simulink model "gm_sampleModel2027_3_sub_sub"  (R2023a)
settings: Solver=VariableStepAuto  StartTime=0.0  StopTime=10.0  RelTol=1e-3
libraries: hdlsllib x5, simulink x2
settings Model: Creator=user1  LastModifiedBy=user1
settings OptimizationCC: BlockReduction=off  ConditionallyExecuteInputs=off
settings DebuggingCC: InheritedTsInSrcMsg=none

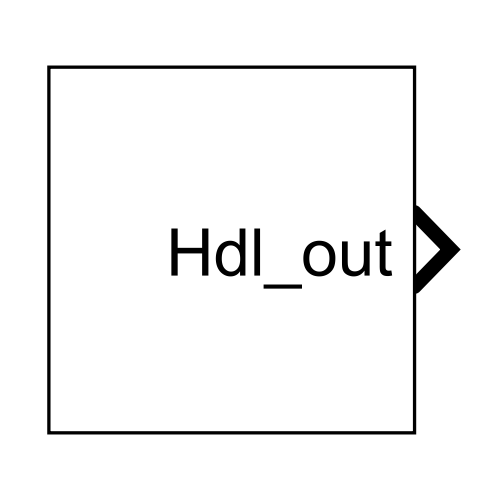
[thumbnail: Simulink's stored preview of the top-level diagram]
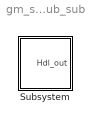
== system gm_sampleModel2027_3_sub_sub ==
  Subsystem : Subsystem

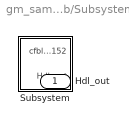
== system gm_sampleModel2027_3_sub_sub/Subsystem ==
  Subsystem : Subsystem
  Hdl_out : Outport  OutDataTypeStr=uint8

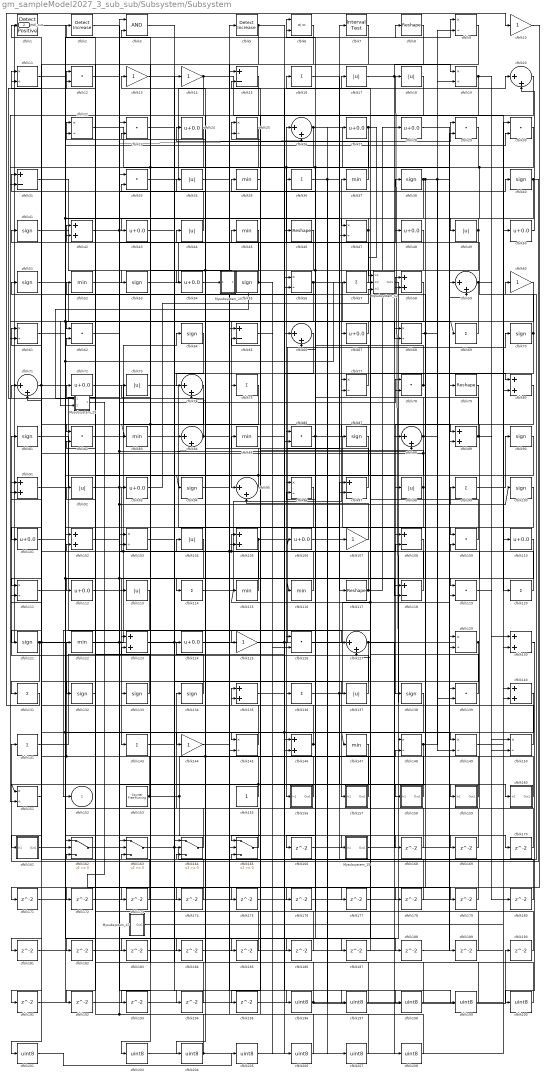
== system gm_sampleModel2027_3_sub_sub/Subsystem/Subsystem ==
  Mysubsystem_15 : Subsystem  TreatAsAtomicUnit=on  RTWFcnName=Mysubsystem_15
      settings: RTWFcnNameOpts=User specified  RTWFileNameOpts=Use function name
  Mysubsystem_19 : Subsystem  TreatAsAtomicUnit=on  RTWFcnName=Mysubsystem_19
      settings: RTWFcnNameOpts=User specified  RTWFileNameOpts=Use function name
  Mysubsystem_29 : Subsystem  TreatAsAtomicUnit=on  RTWFcnName=Mysubsystem_29
      settings: RTWFcnNameOpts=User specified  RTWFileNameOpts=Use function name
  Mysubsystem_47 : Subsystem  TreatAsAtomicUnit=on  RTWFcnName=Mysubsystem_47
      settings: RTWFcnNameOpts=User specified  RTWFileNameOpts=Use function name
  Mysubsystem_52 : Subsystem  TreatAsAtomicUnit=on  RTWFcnName=Mysubsystem_52
      settings: RTWFcnNameOpts=User specified  RTWFileNameOpts=Use function name
  cfblk1 : hdlsllib/Logic and Bit Operations/Detect Rise Positive  vinit=0  OutDataTypeStr=uint8
  cfblk{10,13..14,60,107,125,144} (7 alike) : Gain  OutDataTypeStr=uint8
  cfblk{38,40..41,51,53,55,64,70,81,87,90,94,100,121,132..134,138} (18 alike) : Signum
  cfblk{24,27..28,43,48,50,54,67,72,93,101,106,110,112,124} (15 alike) : Bias  Bias=0.0  SaturateOnIntegerOverflow=off
  cfblk{42,58,80,89,91,102,105,123,130,135,140,146} (12 alike) : Sum  OutDataTypeStr=uint8
  cfblk{9,11,19,22,25,47,56,61,68,77,96,103,111,129,145,148..151} (19 alike) : Product  Inputs=*/  OutDataTypeStr=uint8  RndMeth=Zero  SaturateOnIntegerOverflow=on
  cfblk{17..18,34,44,49,73,92,98,104,113,137} (11 alike) : Abs  OutDataTypeStr=uint8  SaturateOnIntegerOverflow=off
  cfblk{15,31,65,97,108,118} (6 alike) : Sum  Inputs=+-  OutDataTypeStr=uint8
  cfblk{12,23,29..30,33,62,78,82,86,109,119,126,139} (13 alike) : DotProduct  OutDataTypeStr=uint8
  cfblk{16,36,57,69,75,99,114,120,131,136,141,143} (12 alike) : Sum  Inputs=+  OutDataTypeStr=uint8
  cfblk{35,37,45,52,83,85,115..116,122,147} (10 alike) : MinMax  OutDataTypeStr=uint8
  cfblk{8,46,79,117} (4 alike) : Reshape
  cfblk{20,26,59,66,71,74,84,88,95,127} (10 alike) : Sum  Inputs=|++  OutDataTypeStr=uint8
  cfblk153 : hdlsllib/Sources/Counter Free-Running  NumBits=16  tsamp=-1
  cfblk155 : Constant  OutDataTypeStr=uint8  SampleTime=-1
  cfblk156 : Subsystem
      settings: LibrarySourceBlock=|
      | hdlsllib/Ports &
      | Subsystems/Subsystem
  cfblk157 : Subsystem
      settings: LibrarySourceBlock=|
      | hdlsllib/Ports &
      | Subsystems/Subsystem
  cfblk158 : Subsystem
      settings: LibrarySourceBlock=|
      | hdlsllib/Ports &
      | Subsystems/Subsystem
  cfblk159 : Subsystem
      settings: LibrarySourceBlock=|
      | hdlsllib/Ports &
      | Subsystems/Subsystem
  cfblk160 : Subsystem
      settings: LibrarySourceBlock=|
      | hdlsllib/Ports &
      | Subsystems/Subsystem
  cfblk161 : Subsystem
      settings: LibrarySourceBlock=|
      | hdlsllib/Ports &
      | Subsystems/Subsystem
  cfblk{162..165} (4 alike) : Switch  OutDataTypeStr=uint8  SaturateOnIntegerOverflow=off  InputSameDT=off
  cfblk{166,168..195} (29 alike) : Delay  SampleTime=1
  cfblk{196..201,203..208} (12 alike) : DataTypeConversion  OutDataTypeStr=uint8  SaturateOnIntegerOverflow=off  RndMeth=Floor
  cfblk2 : simulink/Logic and Bit Operations/Detect Increase  vinit=0.0  OutDataTypeStr=uint8
      settings: LibrarySourceBlock=|
      | hdlsllib/Logic and Bit
      | Operations/Detect
      | Increase
  cfblk3 : Logic  AllPortsSameDT=off  OutDataTypeStr=boolean
  cfblk5 : simulink/Logic and Bit Operations/Detect Increase  vinit=0.0  OutDataTypeStr=uint8
      settings: LibrarySourceBlock=|
      | hdlsllib/Logic and Bit
      | Operations/Detect
      | Increase
  cfblk6 : RelationalOperator  Operator=<=  OutDataTypeStr=boolean  InputSameDT=off
  cfblk7 : hdlsllib/Logic and Bit Operations/Interval Test  IntervalClosedRight=on  uplimit=0.5  IntervalClosedLeft=on  lowlimit=-0.5  OutDataTypeStr=uint8
  cfblk152 : Outport  OutDataTypeStr=uint8  VectorParamsAs1DForOutWhenUnconnected=off
  Hdl_out : Outport  Port=2  OutDataTypeStr=uint8
  wires:
  cfblk146/1 -> cfblk66/2, cfblk135/1
  cfblk156/1(Out1) -> cfblk71/2, cfblk122/1
  cfblk129/1 -> Hdl_out/1, cfblk157/1(In1)
  cfblk119/1 -> cfblk130/1
  cfblk77/1 -> cfblk51/1
  cfblk56/1 -> cfblk151/2, cfblk152/1
  cfblk33/1 -> cfblk20/1
  cfblk59/1 -> cfblk180/1, cfblk95/1
  cfblk110/1 -> cfblk204/1
  cfblk46/1 -> cfblk156/1(In1)
  cfblk69/1 -> cfblk62/1
  cfblk84/1 -> cfblk198/1, cfblk12/1
  cfblk52/1 -> cfblk194/1, cfblk118/2
  cfblk47/1 -> cfblk43/1, cfblk186/1, cfblk185/1
  cfblk81/1 -> cfblk136/1
  cfblk17/1 -> cfblk19/1, cfblk148/1
  cfblk57/1 -> cfblk26/1
  cfblk132/1 -> cfblk72/1
  cfblk135/1 -> cfblk17/1
  cfblk114/1 -> cfblk37/1
  cfblk31/1 -> cfblk55/1
  cfblk125/1 -> cfblk78/1, cfblk70/1
  cfblk159/1(Out1) -> cfblk25/1
  cfblk26/1 -> cfblk59/1, cfblk181/1, cfblk86/1
  cfblk95/1 -> cfblk94/1, cfblk13/1
  cfblk91/1 -> cfblk33/1
  cfblk105/1 -> cfblk113/1, cfblk7/1
  cfblk98/1 -> cfblk174/1, cfblk61/1, cfblk25/2
  cfblk79/1 -> cfblk138/1
  cfblk106/1 -> cfblk107/1
  cfblk163/1 -> cfblk99/1, cfblk60/1
  cfblk112/1 -> cfblk56/1, cfblk64/1
  cfblk165/1 -> cfblk92/1
  cfblk107/1 -> cfblk95/2
  cfblk164/1 -> cfblk134/1
  cfblk117/1 -> cfblk28/1, cfblk93/1
  cfblk40/1 -> cfblk56/2, cfblk141/1
  cfblk62/1 -> cfblk44/1
  cfblk66/1 -> cfblk86/2
  cfblk73/1 -> cfblk117/1
  cfblk148/1 -> cfblk166/1, cfblk19/2
  cfblk65/1 -> cfblk206/1
  cfblk14/1 -> cfblk61/2, cfblk120/1
  cfblk118/1 -> cfblk67/1
  cfblk151/1 -> cfblk71/1
  cfblk121/1 -> cfblk131/1, cfblk11/2, cfblk58/2
  cfblk137/1 -> cfblk81/1
  cfblk90/1 -> cfblk112/1
  cfblk141/1 -> cfblk46/1
  cfblk136/1 -> cfblk159/1(In1), cfblk18/1
  cfblk20/1 -> cfblk114/1
  cfblk145/1 -> cfblk91/1
  cfblk85/1 -> cfblk197/1, cfblk147/1
  cfblk124/1 -> cfblk106/1, cfblk5/1
  cfblk89/1 -> cfblk150/2, cfblk41/1
  cfblk83/1 -> cfblk14/1
  cfblk157/1(Out1) -> cfblk82/2, cfblk34/1
  cfblk70/1 -> cfblk177/1, cfblk45/1
  cfblk43/1 -> cfblk75/1
  cfblk37/1 -> cfblk24/1
  cfblk42/1 -> cfblk160/1(In1), cfblk40/1
  cfblk153/1 -> cfblk111/2, cfblk208/1, cfblk148/2
  cfblk131/1 -> cfblk10/1
  cfblk139/1 -> cfblk16/1, cfblk115/1
  cfblk100/1 -> cfblk109/1
  cfblk22/1 -> cfblk129/2
  cfblk29/1 -> cfblk173/1, cfblk121/1
  cfblk126/1 -> cfblk79/1
  cfblk12/1 -> cfblk163/1
  cfblk50/1 -> cfblk20/2
  cfblk27/1 -> cfblk165/1, Mysubsystem_52/1(In1)
  cfblk60/1 -> cfblk165/2
  cfblk41/1 -> cfblk53/1
  cfblk30/1 -> cfblk49/1, cfblk31/2, cfblk126/1
  cfblk23/1 -> cfblk96/1
  cfblk120/1 -> cfblk52/1, cfblk105/1
  cfblk138/1 -> cfblk145/1
  cfblk15/1 -> cfblk132/1
  cfblk8/1 -> cfblk105/2
  cfblk102/1 -> cfblk26/2, cfblk88/2
  cfblk161/1(Out1) -> cfblk57/1
  cfblk86/1 -> cfblk176/1, cfblk139/1
  cfblk123/1 -> cfblk168/1, cfblk84/2
  cfblk158/1(Out1) -> cfblk6/1
  cfblk38/1 -> cfblk42/2, cfblk158/1(In1), cfblk59/2, cfblk149/2
  cfblk51/1 -> cfblk146/2
  cfblk36/1 -> cfblk207/1, cfblk118/1
  cfblk150/1 -> cfblk42/1
  cfblk96/1 -> cfblk162/2
  cfblk44/1 -> cfblk31/1
  cfblk49/1 -> cfblk187/1, cfblk47/1
  cfblk122/1 -> cfblk108/2, cfblk68/1
  cfblk53/1 -> cfblk38/1
  cfblk82/1 -> cfblk87/1
  cfblk88/1 -> cfblk193/1, cfblk9/2, cfblk35/1
  cfblk71/1 -> cfblk111/1, cfblk116/1, cfblk188/1, cfblk145/2
  cfblk101/1 -> cfblk9/1
  cfblk25/1 -> cfblk144/1
  cfblk1/1 -> cfblk47/2, cfblk69/1, cfblk97/2
  cfblk34/1 -> cfblk80/1
  cfblk134/1 -> cfblk124/1
  cfblk108/1 -> cfblk143/1
  cfblk144/1 -> cfblk29/1
  cfblk104/1 -> cfblk164/2
  cfblk74/1 -> cfblk101/1
  cfblk143/1 -> cfblk48/1
  cfblk149/1 -> cfblk50/1
  cfblk99/1 -> cfblk90/1
  cfblk72/1 -> cfblk89/1
  cfblk35/1 -> cfblk15/2
  cfblk160/1(Out1) -> cfblk58/1
  cfblk97/1 -> cfblk22/1
  cfblk162/1 -> cfblk8/1, cfblk100/1
  cfblk55/1 -> cfblk126/2, cfblk33/2
  cfblk45/1 -> cfblk54/1
  cfblk155/1 -> cfblk151/1, cfblk23/2
  cfblk5/1 -> cfblk68/2, cfblk83/1, cfblk133/1
  cfblk9/1 -> cfblk82/1
  cfblk133/1 -> cfblk102/2
  cfblk92/1 -> cfblk78/2, cfblk127/1
  cfblk19/1 -> cfblk150/1, cfblk103/2
  cfblk80/1 -> cfblk119/1
  cfblk109/1 -> cfblk77/1
  cfblk48/1 -> cfblk74/2, cfblk123/1
  cfblk64/1 -> cfblk74/1
  cfblk13/1 -> cfblk137/1
  cfblk18/1 -> cfblk125/1
  cfblk116/1 -> cfblk73/1
  cfblk58/1 -> cfblk91/2
  cfblk54/1 -> cfblk149/1
  cfblk3/1 -> cfblk196/1
  cfblk111/1 -> cfblk30/2, Mysubsystem_52/2(In2)
  cfblk127/1 -> cfblk169/1, cfblk161/1(In1)
  cfblk16/1 -> cfblk98/1
  cfblk68/1 -> cfblk139/2, cfblk108/1
  cfblk78/1 -> cfblk178/1, cfblk36/1
  cfblk115/1 -> cfblk11/1
  cfblk166/1 -> cfblk88/1
  cfblk168/1 -> cfblk102/1
  cfblk169/1 -> cfblk123/2
  cfblk11/1 -> cfblk170/1
  cfblk170/1 -> cfblk109/2
  cfblk10/1 -> cfblk171/1
  cfblk171/1 -> cfblk146/1
  cfblk24/1 -> cfblk172/1
  cfblk172/1 -> cfblk29/2
  cfblk173/1 -> cfblk162/3
  cfblk174/1 -> cfblk164/3
  cfblk175/1 -> cfblk135/2
  cfblk176/1 -> cfblk96/2
  cfblk177/1 -> cfblk127/2
  cfblk178/1 -> cfblk12/2
  cfblk94/1 -> cfblk179/1
  cfblk179/1 -> cfblk97/1
  cfblk180/1 -> cfblk1/1
  cfblk181/1 -> cfblk130/2
  cfblk87/1 -> cfblk182/1
  cfblk182/1 -> cfblk84/1
  cfblk183/1 -> cfblk89/2
  cfblk75/1 -> cfblk184/1
  cfblk184/1 -> cfblk30/1
  cfblk185/1 -> cfblk163/2
  cfblk186/1 -> cfblk163/3
  cfblk187/1 -> cfblk77/2
  cfblk188/1 -> cfblk119/2
  cfblk28/1 -> cfblk189/1
  cfblk189/1 -> cfblk22/2
  cfblk190/1 -> cfblk6/2
  cfblk7/1 -> cfblk191/1
  cfblk191/1 -> cfblk162/1
  cfblk113/1 -> cfblk192/1
  cfblk192/1 -> cfblk15/1
  cfblk193/1 -> cfblk80/2
  cfblk194/1 -> cfblk164/1
  cfblk147/1 -> cfblk195/1
  cfblk195/1 -> cfblk85/1
  cfblk196/1 -> cfblk165/3, cfblk27/1, cfblk190/1
  cfblk197/1 -> cfblk3/1
  cfblk198/1 -> cfblk3/2
  cfblk2/1 -> cfblk199/1
  cfblk199/1 -> cfblk104/1
  cfblk130/1 -> cfblk200/1
  cfblk200/1 -> cfblk2/1
  cfblk140/1 -> cfblk201/1
  cfblk6/1 -> cfblk203/1
  cfblk203/1 -> cfblk140/2
  cfblk204/1 -> cfblk23/1, cfblk66/1
  cfblk201/1 -> cfblk205/1
  cfblk205/1 -> cfblk110/1
  cfblk206/1 -> cfblk103/1, cfblk62/2
  cfblk207/1 -> cfblk65/1
  cfblk208/1 -> cfblk65/2
  cfblk103/1 -> Mysubsystem_15/1(In1)
  Mysubsystem_15/1(Out1) -> cfblk129/1
  cfblk61/1 -> Mysubsystem_19/1(In1)
  Mysubsystem_19/1(Out1) -> Mysubsystem_29/1(In1)
  cfblk67/1 -> Mysubsystem_29/2(In2)
  Mysubsystem_29/1(Out1) -> cfblk175/1
  Mysubsystem_47/1(Out1) -> cfblk140/1
  cfblk93/1 -> Mysubsystem_52/3(In3)
  Mysubsystem_52/1(Out1) -> cfblk183/1

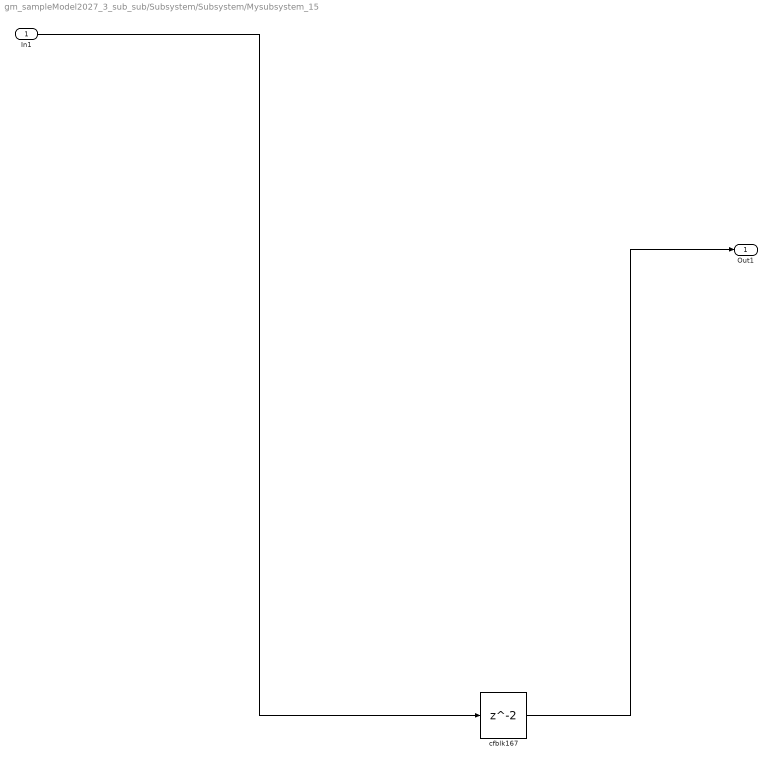
== system gm_sampleModel2027_3_sub_sub/Subsystem/Subsystem/Mysubsystem_15 ==
  In1 : Inport
  cfblk167 : Delay  SampleTime=1
  Out1 : Outport
  wires:
  cfblk167/1 -> Out1/1
  In1/1 -> cfblk167/1

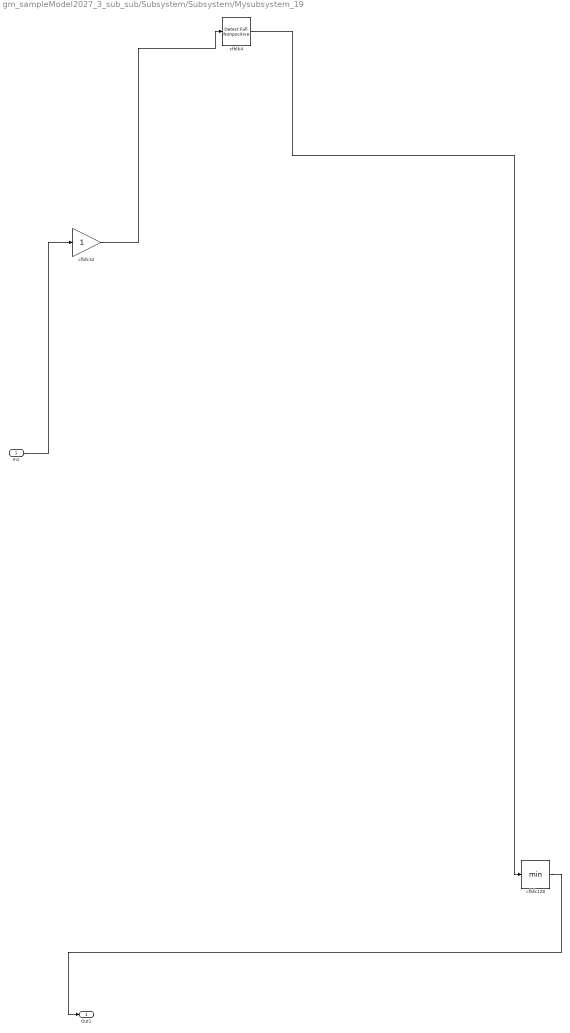
== system gm_sampleModel2027_3_sub_sub/Subsystem/Subsystem/Mysubsystem_19 ==
  In1 : Inport
  cfblk128 : MinMax
  cfblk32 : Gain
  cfblk4 : hdlsllib/Logic and Bit Operations/Detect Fall Nonpositive  vinit=0  OutDataTypeStr=boolean
  Out1 : Outport
  wires:
  cfblk128/1 -> Out1/1
  In1/1 -> cfblk32/1
  cfblk32/1 -> cfblk4/1
  cfblk4/1 -> cfblk128/1

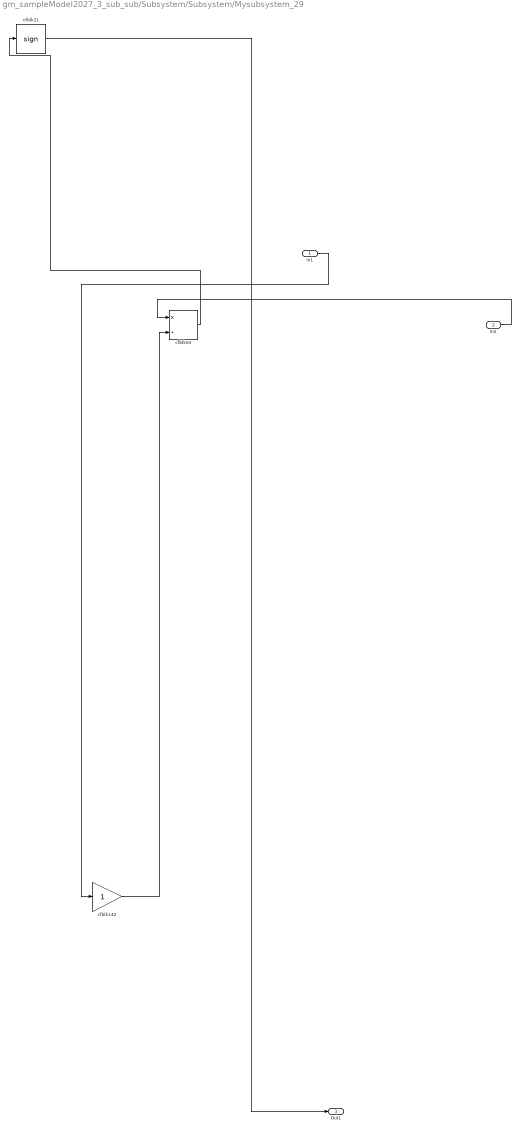
== system gm_sampleModel2027_3_sub_sub/Subsystem/Subsystem/Mysubsystem_29 ==
  In1 : Inport
  In2 : Inport  Port=2
  cfblk142 : Gain
  cfblk21 : Signum
  cfblk63 : Product  Inputs=*/  RndMeth=Zero  SaturateOnIntegerOverflow=on
  Out1 : Outport
  wires:
  In2/1 -> cfblk63/1
  In1/1 -> cfblk142/1
  cfblk63/1 -> cfblk21/1
  cfblk142/1 -> cfblk63/2
  cfblk21/1 -> Out1/1

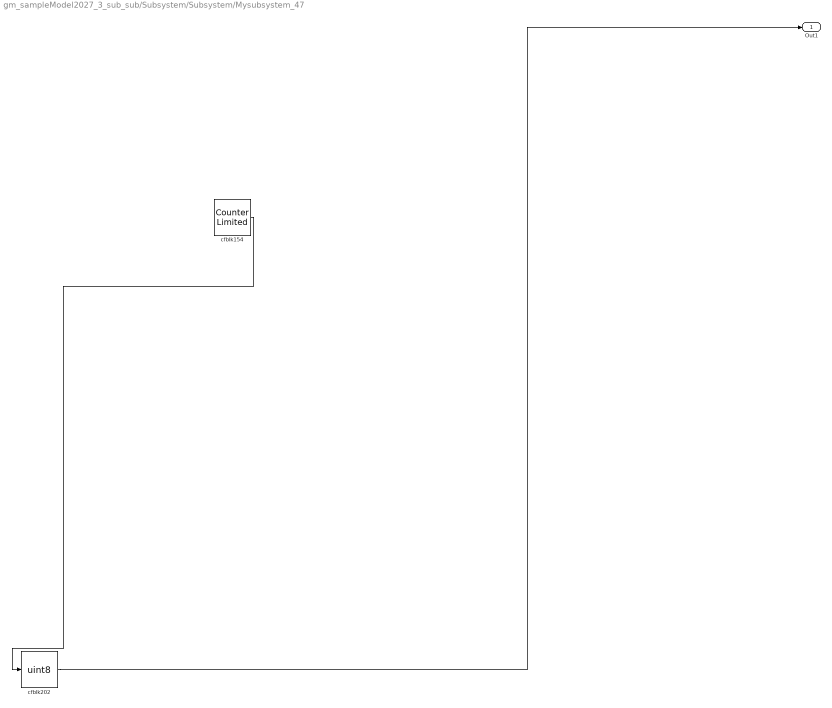
== system gm_sampleModel2027_3_sub_sub/Subsystem/Subsystem/Mysubsystem_47 ==
  cfblk154 : hdlsllib/Sources/Counter Limited  uplimit=7  tsamp=-1
  cfblk202 : DataTypeConversion  OutDataTypeStr=uint8  SaturateOnIntegerOverflow=off  RndMeth=Floor
  Out1 : Outport
  wires:
  cfblk202/1 -> Out1/1
  cfblk154/1 -> cfblk202/1

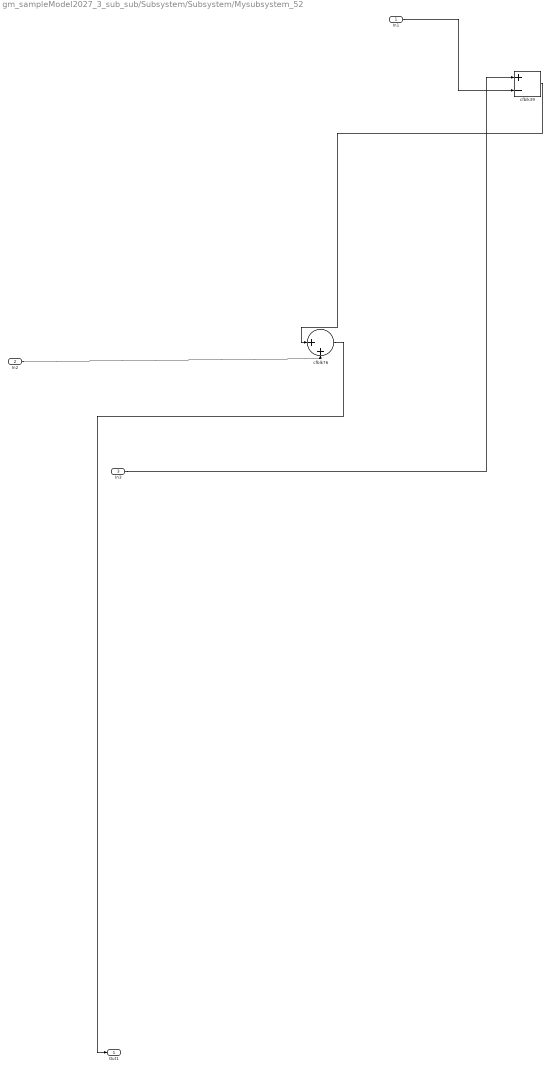
== system gm_sampleModel2027_3_sub_sub/Subsystem/Subsystem/Mysubsystem_52 ==
  In1 : Inport
  In2 : Inport  Port=2
  In3 : Inport  Port=3
  cfblk39 : Sum  Inputs=+-
  cfblk76 : Sum  Inputs=|++
  Out1 : Outport
  wires:
  In1/1 -> cfblk39/2
  cfblk76/1 -> Out1/1
  In2/1 -> cfblk76/2
  In3/1 -> cfblk39/1
  cfblk39/1 -> cfblk76/1

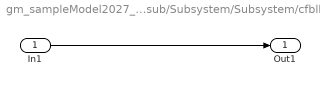
== system gm_sampleModel2027_3_sub_sub/Subsystem/Subsystem/cfblk156 ==
  In1 : Inport
  Out1 : Outport
  wires:
  In1/1 -> Out1/1

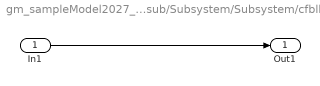
== system gm_sampleModel2027_3_sub_sub/Subsystem/Subsystem/cfblk157 ==
  In1 : Inport
  Out1 : Outport
  wires:
  In1/1 -> Out1/1

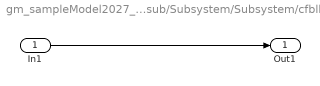
== system gm_sampleModel2027_3_sub_sub/Subsystem/Subsystem/cfblk158 ==
  In1 : Inport
  Out1 : Outport
  wires:
  In1/1 -> Out1/1

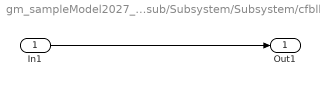
== system gm_sampleModel2027_3_sub_sub/Subsystem/Subsystem/cfblk159 ==
  In1 : Inport
  Out1 : Outport
  wires:
  In1/1 -> Out1/1

== system gm_sampleModel2027_3_sub_sub/Subsystem/Subsystem/cfblk160 ==
  In1 : Inport
  Out1 : Outport
  wires:
  In1/1 -> Out1/1

== system gm_sampleModel2027_3_sub_sub/Subsystem/Subsystem/cfblk161 ==
  In1 : Inport
  Out1 : Outport
  wires:
  In1/1 -> Out1/1
